simulink model "Simulazione"  (R2023a)
settings: Solver=FixedStepAuto  StartTime=0.0  StopTime=10.0  FixedStep=Tc_sim  RelTol=1e-3
undefined symbols (not defined in the file): a, A_sim, b, B_sim, C, k_m_sim, R_m_sim, X0
settings Model: Creator=ricca  LastModifiedBy=ricca
settings DebuggingCC: AlgebraicLoopMsg=none

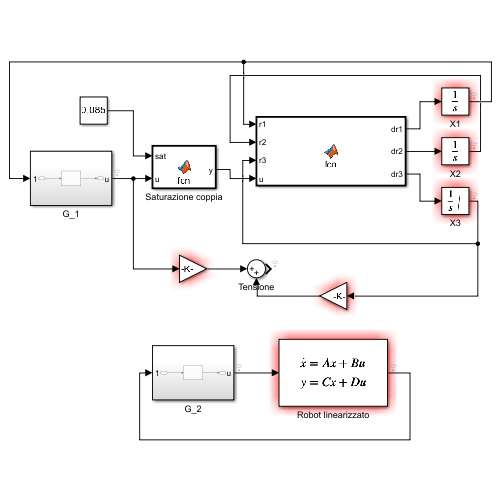
[thumbnail: Simulink's stored preview of the top-level diagram]
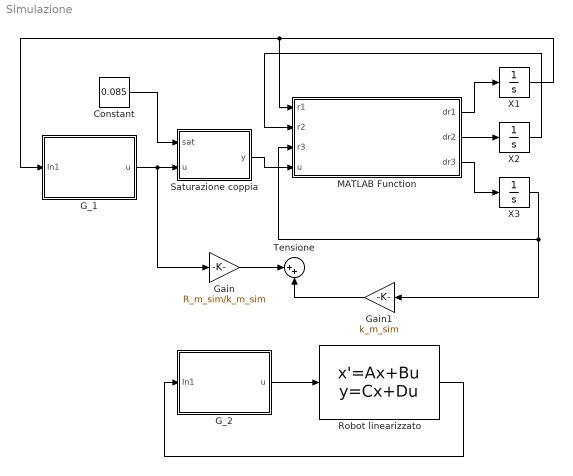
== system Simulazione ==
  Constant : Constant  Value=0.085
  G_1 : Subsystem
  G_2 : Subsystem
  Gain : Gain  Gain=R_m_sim/k_m_sim
  Gain1 : Gain  Gain=k_m_sim
  MATLAB Function : MATLAB Function  TreatAsAtomicUnit=on
  Robot linearizzato : StateSpace  A=A_sim  B=B_sim  C=C  D=0  InitialCondition=X0
  Saturazione coppia : MATLAB Function  TreatAsAtomicUnit=on
  Tensione : Sum  Inputs=|++
  X1 : Integrator  InitialCondition=X0(1)
  X2 : Integrator  InitialCondition=X0(2)
  X3 : Integrator  InitialCondition=X0(3)  LimitOutput=on  UpperSaturationLimit=41.8  LowerSaturationLimit=-41.8
  wires:
  Robot linearizzato/1 -> G_2/1(In1)
  MATLAB Function/1(dr1) -> X1/1
  MATLAB Function/2(dr2) -> X2/1
  MATLAB Function/3(dr3) -> X3/1
  X1/1 -> MATLAB Function/1(r1), G_1/1(In1)
  G_2/1(u) -> Robot linearizzato/1
  G_1/1(u) -> Gain/1, Saturazione coppia/2(u)
  X2/1 -> MATLAB Function/2(r2)
  X3/1 -> Gain1/1, MATLAB Function/3(r3)
  Gain/1 -> Tensione/1
  Gain1/1 -> Tensione/2
  Saturazione coppia/1(y) -> MATLAB Function/4(u)
  Constant/1 -> Saturazione coppia/1(sat)

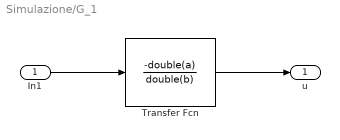
== system Simulazione/G_1 ==
  In1 : Inport
  Transfer Fcn : TransferFcn  Numerator=-double(a)  Denominator=double(b)
  u : Outport
  wires:
  In1/1 -> Transfer Fcn/1
  Transfer Fcn/1 -> u/1

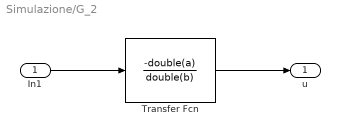
== system Simulazione/G_2 ==
  In1 : Inport
  Transfer Fcn : TransferFcn  Numerator=-double(a)  Denominator=double(b)
  u : Outport
  wires:
  In1/1 -> Transfer Fcn/1
  Transfer Fcn/1 -> u/1

== matlab function Simulazione/Saturazione coppia ==
  data: sat input; u input; y output
function y = fcn(sat,u)
if(abs(u) <= sat)
    y=u;
else
    y=u/abs(u)*sat;
end

== matlab function Simulazione/MATLAB Function ==
  data: dr1 output; r1 input; r2 input; r3 input; u input; dr2 output; dr3 output
function [dr1,dr2,dr3]=fcn(r1,r2,r3,u)
%#codegen
g=9.81; %m/s^2
M_T=267e-3; %Kg
T_cm=86.8e-3; %m
Ir_cm_M=135.2e-6; %Kg*m^2
R_R=(52e-3)/2; %m
Mm=(100e-3)*2+(24e-3); %Kg, massa motori
Mr=(17e-3)*2; %Kg, massa ruote
I_TOT=(Mr/2)*R_R^2+R_R^2*(Mr+M_T+Mm); %Kg*m^2
I_TR=Ir_cm_M+M_T*T_cm^2; %Kg*m^2
b=0.89; %1/s
k_m=12;
R_m=2.41;

dr1=r2;
dr2=-(I_TR*b*r2 - M_T*T_cm*g*sin(r1) + (M_T*R_R*T_cm*cos(r1)*(M_T*R_R*T_cm*sin(r1)*r2^2 + u - I_TOT*b*r3))/I_TOT)/(I_TR - (M_T^2*R_R^2*T_cm^2*cos(r1)^2)/I_TOT);
dr3=(u - I_TOT*b*r3 + M_T*R_R*T_cm*r2^2*sin(r1) + (M_T*R_R*T_cm*cos(r1)*(I_TR*b*r2 - M_T*T_cm*g*sin(r1) + (M_T*R_R*T_cm*cos(r1)*(M_T*R_R*T_cm*sin(r1)*r2^2 + u - I_TOT*b*r3))/I_TOT))/(I_TR - (M_T^2*R_R^2*T_cm^2*cos(r1)^2)/I_TOT))/I_TOT;
